simulink model "Chap6_RealPassband_rcos"  (R2015a)
settings: Solver=VariableStepDiscrete  StartTime=0.0  StopTime=1  RelTol=1e-3
InitFcn:
  | clear
  | BitRate = 4e6;
  | M = 16;
  | l = log2(M);
  | SymbolRate = BitRate / l;
  | UpsampleTimes = 8;
  | SampleRate = SymbolRate * UpsampleTimes;
  | Fc = 2.5e6;
  | Fs = SampleRate;
  | SamplePerFrame = 4000;
  | SymbolPerFrame = SamplePerFrame / l;
  | 
  | SNR = 10;
  | 
  | EsN0 = SNR + 10 * log10(UpsampleTimes);
  | EbN0 = EsN0 - 10 * log10(l);
  | BERBaseBandTheory = berawgn(EbN0, 'qam', M);
  | 
  | EsN0 = SNR + 10 * log10(UpsampleTimes / 2);
  | EbN0 = EsN0 - 10 * log10(l);
  | BERPassBandTheory = berawgn(EbN0, 'qam', M);
libraries: commfilt2 x4, commdigbbndam3 x3, commchan3 x2, dspsrcs4 x2, commsink2 x2, commrandsrc2 x1
settings Model: Creator=Administrator  LastModifiedBy=Administrator
settings DebuggingCC: SignalRangeChecking=warning  ParameterOverflowMsg=warning  ParameterPrecisionLossMsg=none  ParameterTunabilityLossMsg=none
settings HardwareCC: ProdHWDeviceType=ASIC/FPGA->ASIC/FPGA  TargetHWDeviceType=Generic->Custom  ProdEqTarget=off

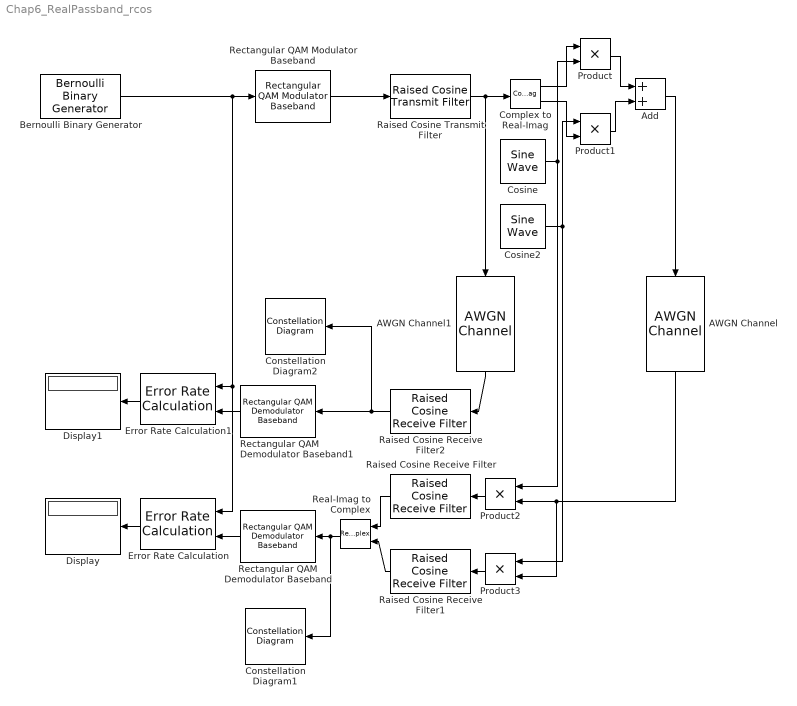
== system Chap6_RealPassband_rcos ==
  AWGN Channel : commchan3/AWGN Channel  InputProcessing=Columns as channels (frame based)  seed=67  noiseMode="Signal to noise ratio  (SNR)"  EbNodB=10  EsNodB=10  SNRdB=SNR  bitsPerSym=4  Ps=1  Tsym=4e-6  variance=1
  AWGN Channel1 : commchan3/AWGN Channel  InputProcessing=Columns as channels (frame based)  seed=67  noiseMode="Signal to noise ratio  (SNR)"  EbNodB=10  EsNodB=10  SNRdB=SNR  bitsPerSym=4  Ps=1  Tsym=4e-6  variance=1
  Add : Sum
  Bernoulli Binary Generator : commrandsrc2/Bernoulli Binary Generator  P=0.5  seed=61  Ts=1/BitRate  frameBased=on  sampPerFrame=SamplePerFrame  orient=off  outDataType=double
  Complex to Real-Imag : ComplexToRealImag
  Constellation Diagram1 : ConstellationDiagram
  Constellation Diagram2 : ConstellationDiagram
  Cosine : dspsrcs4/Sine Wave  Amplitude=sqrt(2)  Frequency=Fc  Phase=pi/2  SampleMode=Discrete  OutComplex=Real  CompMethod=Trigonometric fcn  TableSize=Speed  SampleTime=1/Fs  SamplesPerFrame=SymbolPerFrame * UpsampleTimes  ResetState=Restart at time zero  dataType=double  wordLen=16  udDataType=sfix(16)  fracBitsMode=Best precision  numFracBits=15  OutDataTypeStr=double  LastOutDataTypeStr=double
  Cosine2 : dspsrcs4/Sine Wave  Amplitude=sqrt(2)  Frequency=Fc  Phase=0  SampleMode=Discrete  OutComplex=Real  CompMethod=Trigonometric fcn  TableSize=Speed  SampleTime=1/Fs  SamplesPerFrame=SymbolPerFrame * UpsampleTimes  ResetState=Restart at time zero  dataType=double  wordLen=16  udDataType=sfix(16)  fracBitsMode=Best precision  numFracBits=15  OutDataTypeStr=double  LastOutDataTypeStr=double
  Display : Display
  Display1 : Display
  Error Rate Calculation : commsink2/Error Rate Calculation  N=5 * UpsampleTimes  st_delay=0  cp_mode=Entire frame  subframe=[]  PMode=Port  WsName=ErrorVec  RsMode2=off  stop=off  numErr=100  maxBits=1e6
  Error Rate Calculation1 : commsink2/Error Rate Calculation  N=5 * UpsampleTimes  st_delay=0  cp_mode=Entire frame  subframe=[]  PMode=Port  WsName=ErrorVec  RsMode2=off  stop=off  numErr=100  maxBits=1e6
  Product{,1..3} (4 alike) : Product  RndMeth=Zero
  Raised Cosine Receive Filter : commfilt2/Raised Cosine Receive Filter  filtType=Square root  N=UpsampleTimes  filtSpan=10  currentFiltSpan=10  D=5  R=0.2  sampMode=Mute  saveAsFlag=0  rateMode=Downsampling  downFactor=UpsampleTimes  downOffset=0  framing=Enforce single-rate processing  InputProcessing=Columns as channels (frame based)  checkGain=Normalized  filterGain=1/sqrt(UpsampleTimes)  checkCoeff=off  variableName=rcRxFilt  launchFVT=on  roundingMode=Floor  overflowMode=off
  Raised Cosine Receive Filter1 : commfilt2/Raised Cosine Receive Filter  filtType=Square root  N=UpsampleTimes  filtSpan=10  currentFiltSpan=10  D=5  R=0.2  sampMode=Mute  saveAsFlag=0  rateMode=Downsampling  downFactor=UpsampleTimes  downOffset=0  framing=Enforce single-rate processing  InputProcessing=Columns as channels (frame based)  checkGain=Normalized  filterGain=1/sqrt(UpsampleTimes)  checkCoeff=off  variableName=rcRxFilt1  launchFVT=on  roundingMode=Floor  overflowMode=off
  Raised Cosine Receive Filter2 : commfilt2/Raised Cosine Receive Filter  filtType=Square root  N=UpsampleTimes  filtSpan=10  currentFiltSpan=10  D=5  R=0.2  sampMode=Mute  saveAsFlag=0  rateMode=Downsampling  downFactor=UpsampleTimes  downOffset=0  framing=Enforce single-rate processing  InputProcessing=Columns as channels (frame based)  checkGain=Normalized  filterGain=1/sqrt(UpsampleTimes)  checkCoeff=off  variableName=rcRxFilt2  launchFVT=on  roundingMode=Floor  overflowMode=off
  Raised Cosine Transmit Filter : commfilt2/Raised Cosine Transmit Filter  filtType=Square root  filtSpan=10  currentFiltSpan=10  D=5  R=0.2  sampMode=Mute  saveAsFlag=0  N=UpsampleTimes  framing=Enforce single-rate processing  InputProcessing=Columns as channels (frame based)  checkGain=Normalized  filterGain=sqrt(UpsampleTimes)  checkCoeff=off  variableName=rcTxFilt  launchFVT=on  roundingMode=Floor  overflowMode=off
  Real-Imag to Complex : RealImagToComplex
  Rectangular QAM Demodulator Baseband : commdigbbndam3/Rectangular QAM Demodulator Baseband  M=16  PowType=Average Power  MinDist=2  AvgPow=1  PeakPow=1  Ph=0  Dec=Gray  Mapping=[0:15]  OutType=Bit  DecType=Hard decision  VarSource=Dialog  Variance=1  outDtype1=Inherit via internal rule  outDtype2=Inherit via internal rule  derotateFactorWordLen=16  denormFactorWordLen=16  prodOutWordLen=32  prodOutRoundingMode=Floor  prodOutOverflowMode=Wrap  sumWordLen=32
  Rectangular QAM Demodulator Baseband1 : commdigbbndam3/Rectangular QAM Demodulator Baseband  M=16  PowType=Average Power  MinDist=2  AvgPow=1  PeakPow=1  Ph=0  Dec=Gray  Mapping=[0:15]  OutType=Bit  DecType=Hard decision  VarSource=Dialog  Variance=1  outDtype1=Inherit via internal rule  outDtype2=Inherit via internal rule  derotateFactorWordLen=16  denormFactorWordLen=16  prodOutWordLen=32  prodOutRoundingMode=Floor  prodOutOverflowMode=Wrap  sumWordLen=32
  Rectangular QAM Modulator Baseband : commdigbbndam3/Rectangular QAM Modulator Baseband  M=M  InType=Bit  Enc=Gray  Mapping=[0:15]  PowType=Average Power  MinDist=2  AvgPow=1  PeakPow=1  Ph=0  outDtype=double  outWordLen=16  outUDDataType=sfix(16)  outFracLenMode=Best precision  outFracLen=15
  wires:
  Bernoulli Binary Generator/1 -> Error Rate Calculation1/1, Error Rate Calculation/1, Rectangular QAM Modulator Baseband/1
  Add/1 -> AWGN Channel/1
  Rectangular QAM Modulator Baseband/1 -> Raised Cosine Transmit Filter/1
  Product1/1 -> Add/2
  Product/1 -> Add/1
  Complex to Real-Imag/1 -> Product/1
  Complex to Real-Imag/2 -> Product1/2
  Raised Cosine Transmit Filter/1 -> Complex to Real-Imag/1, AWGN Channel1/1
  Cosine/1 -> Product2/1, Product/2
  Cosine2/1 -> Product3/1, Product1/1
  AWGN Channel/1 -> Product3/2, Product2/2
  Product2/1 -> Raised Cosine Receive Filter/1
  Product3/1 -> Raised Cosine Receive Filter1/1
  Raised Cosine Receive Filter/1 -> Real-Imag to Complex/1
  Raised Cosine Receive Filter1/1 -> Real-Imag to Complex/2
  Real-Imag to Complex/1 -> Rectangular QAM Demodulator Baseband/1, Constellation Diagram1/1
  Rectangular QAM Demodulator Baseband/1 -> Error Rate Calculation/2
  Error Rate Calculation/1 -> Display/1
  AWGN Channel1/1 -> Raised Cosine Receive Filter2/1
  Raised Cosine Receive Filter2/1 -> Constellation Diagram2/1, Rectangular QAM Demodulator Baseband1/1
  Rectangular QAM Demodulator Baseband1/1 -> Error Rate Calculation1/2
  Error Rate Calculation1/1 -> Display1/1
